simulink model "21-E"  (R2014a)
settings: Solver=FixedStepDiscrete  StartTime=0.0  StopTime=10.0  FixedStep=0.0005  RelTol=1e-3
undefined symbols (not defined in the file): add_k1_100, add_k2_100, ADDspeed, cal_acc_div, cal_acc_flo_add, cal_acc_min, cal_an_div, cal_an_min, cal_bre_div, cal_bre_en_add, cal_bre_flo_add, cal_bre_min, cal_conf_off, cal_conf_on, controller, ecucoder_acal, enres_on_add, enres_per_add
libraries: simulink x165, ec55xxlib x29
(part 5 of 6)

== system 21-E/run/ctrl/ECU_1L/ctrl_1L ==
  ctrl_1L : Inport
  BitCov : DataTypeConversion  OutDataTypeStr=uint8
  Constant{3..8} (6 alike) : Constant  Value=0  OutDataTypeStr=uint8
  ctrl_1LCOV : DataTypeConversion  OutDataTypeStr=uint8
  ctrl_1LRon : Rounding  Operator=round
  ctrl_1L_1sat : Saturate  UpperLimit=65535  LowerLimit=0
  ctrl_1L_And : simulink/Logic and Bit Operations/Bitwise Operator  logicop=AND  UseBitMask=off  NumInputPorts=2  BitMask=bin2dec('11011001')  BitMaskRealWorld=Stored Integer
  ctrl_1L_And_C : Constant  Value=255  OutDataTypeStr=uint32
  ctrl_1L_Convert : DataTypeConversion  OutDataTypeStr=uint32
  ctrl_1L_D : Product  Inputs=*/
  ctrl_1L_D1 : Product  Inputs=*/
  ctrl_1L_F : Constant  OutDataTypeStr=single
  ctrl_1L_L : simulink/Logic and Bit Operations/Bitwise Operator  logicop=AND  UseBitMask=on  BitMask=65535  BitMaskRealWorld=Stored Integer
  ctrl_1L_O : Constant  Value=0  OutDataTypeStr=single
  ctrl_1L_S : ArithShift
  ctrl_1L_sat : Saturate  UpperLimit=65535  LowerLimit=0
  ctrl_1L_st : Sum  Inputs=+-
  ctrl_1Loutput2_C : Constant  Value=256
  output1 : Outport
  output2 : Outport  Port=2
  output3 : Outport  Port=3
  output4 : Outport  Port=4
  output5 : Outport  Port=5
  output6 : Outport  Port=6
  output7 : Outport  Port=7
  output8 : Outport  Port=8
  wires:
  Constant8/1 -> output8/1
  Constant7/1 -> output7/1
  Constant6/1 -> output6/1
  Constant5/1 -> output5/1
  Constant4/1 -> output4/1
  Constant3/1 -> output3/1
  BitCov/1 -> output1/1
  ctrl_1L_And/1 -> BitCov/1
  ctrl_1L_And_C/1 -> ctrl_1L_And/2
  ctrl_1LCOV/1 -> output2/1
  ctrl_1L_D1/1 -> ctrl_1LCOV/1
  ctrl_1Loutput2_C/1 -> ctrl_1L_D1/2
  ctrl_1L_L/1 -> ctrl_1L_And/1, ctrl_1L_D1/1
  ctrl_1L_Convert/1 -> ctrl_1L_L/1
  ctrl_1L_1sat/1 -> ctrl_1L_Convert/1
  ctrl_1L_S/1 -> ctrl_1L_1sat/1
  ctrl_1LRon/1 -> ctrl_1L_S/1
  ctrl_1L_D/1 -> ctrl_1LRon/1
  ctrl_1L_F/1 -> ctrl_1L_D/2
  ctrl_1L_st/1 -> ctrl_1L_D/1
  ctrl_1L_O/1 -> ctrl_1L_st/2
  ctrl_1L_sat/1 -> ctrl_1L_st/1
  ctrl_1L/1 -> ctrl_1L_sat/1

== system 21-E/run/ctrl/ECU_1L/max_n ==
  max_n : Inport
  BitCov : DataTypeConversion  OutDataTypeStr=uint8
  Constant{1..2,5..8} (6 alike) : Constant  Value=0  OutDataTypeStr=uint8
  max_nABS : Abs
  max_nCOV : DataTypeConversion  OutDataTypeStr=uint8
  max_nCS : ArithShift  BitShiftNumber=-16
  max_nConS : Constant  OutDataTypeStr=single
  max_nCosR : Constant  Value=0  OutDataTypeStr=uint8
  max_nROP : RelationalOperator  Operator=<  OutDataTypeStr=boolean
  max_nRon : Rounding  Operator=round
  max_nSW : Switch  Criteria=u2 ~= 0
  max_n_1sat : Saturate  UpperLimit=65535  LowerLimit=0
  max_n_And : simulink/Logic and Bit Operations/Bitwise Operator  logicop=AND  UseBitMask=off  NumInputPorts=2  BitMask=bin2dec('11011001')  BitMaskRealWorld=Stored Integer
  max_n_And_C : Constant  Value=255  OutDataTypeStr=uint32
  max_n_Convert : DataTypeConversion  OutDataTypeStr=uint32
  max_n_D : Product  Inputs=*/
  max_n_D1 : Product  Inputs=*/
  max_n_F : Constant  OutDataTypeStr=single
  max_n_L : simulink/Logic and Bit Operations/Bitwise Operator  logicop=AND  UseBitMask=on  BitMask=65535  BitMaskRealWorld=Stored Integer
  max_n_O : Constant  Value=0  OutDataTypeStr=single
  max_n_S : ArithShift
  max_n_sat : Saturate  UpperLimit=32767  LowerLimit=-32768
  max_n_st : Sum  Inputs=+-
  max_noutput4_C : Constant  Value=256
  max_nsubcon : Sum  Inputs=+-
  output1 : Outport
  output2 : Outport  Port=2
  output3 : Outport  Port=3
  output4 : Outport  Port=4
  output5 : Outport  Port=5
  output6 : Outport  Port=6
  output7 : Outport  Port=7
  output8 : Outport  Port=8
  wires:
  Constant8/1 -> output8/1
  Constant7/1 -> output7/1
  Constant6/1 -> output6/1
  Constant5/1 -> output5/1
  Constant2/1 -> output2/1
  Constant1/1 -> output1/1
  BitCov/1 -> output3/1
  max_n_And/1 -> BitCov/1
  max_n_And_C/1 -> max_n_And/2
  max_nCOV/1 -> output4/1
  max_n_D1/1 -> max_nCOV/1
  max_noutput4_C/1 -> max_n_D1/2
  max_n_L/1 -> max_n_And/1, max_n_D1/1
  max_n_Convert/1 -> max_n_L/1
  max_n_1sat/1 -> max_n_Convert/1
  max_n_S/1 -> max_n_1sat/1
  max_nSW/1 -> max_n_S/1
  max_nROP/1 -> max_nSW/2
  max_nsubcon/1 -> max_nSW/1
  max_nABS/1 -> max_nsubcon/2
  max_nCS/1 -> max_nsubcon/1
  max_nConS/1 -> max_nCS/1
  max_nCosR/1 -> max_nROP/2
  max_nRon/1 -> max_nSW/3, max_nABS/1, max_nROP/1
  max_n_D/1 -> max_nRon/1
  max_n_F/1 -> max_n_D/2
  max_n_st/1 -> max_n_D/1
  max_n_O/1 -> max_n_st/2
  max_n_sat/1 -> max_n_st/1
  max_n/1 -> max_n_sat/1

== system 21-E/run/ctrl/ECU_1R/TN_1R ==
  TN_1R : Inport
  BitCov : DataTypeConversion  OutDataTypeStr=uint8
  Constant{1..6} (6 alike) : Constant  Value=0  OutDataTypeStr=uint8
  TN_1RABS : Abs
  TN_1RCOV : DataTypeConversion  OutDataTypeStr=uint8
  TN_1RCS : ArithShift  BitShiftNumber=-16
  TN_1RConS : Constant  OutDataTypeStr=single
  TN_1RCosR : Constant  Value=0  OutDataTypeStr=uint8
  TN_1RROP : RelationalOperator  Operator=<  OutDataTypeStr=boolean
  TN_1RRon : Rounding  Operator=round
  TN_1RSW : Switch  Criteria=u2 ~= 0
  TN_1R_1sat : Saturate  UpperLimit=65535  LowerLimit=0
  TN_1R_And : simulink/Logic and Bit Operations/Bitwise Operator  logicop=AND  UseBitMask=off  NumInputPorts=2  BitMask=bin2dec('11011001')  BitMaskRealWorld=Stored Integer
  TN_1R_And_C : Constant  Value=255  OutDataTypeStr=uint32
  TN_1R_Convert : DataTypeConversion  OutDataTypeStr=uint32
  TN_1R_D : Product  Inputs=*/
  TN_1R_D1 : Product  Inputs=*/
  TN_1R_F : Constant  OutDataTypeStr=single
  TN_1R_L : simulink/Logic and Bit Operations/Bitwise Operator  logicop=AND  UseBitMask=on  BitMask=65535  BitMaskRealWorld=Stored Integer
  TN_1R_O : Constant  Value=0  OutDataTypeStr=single
  TN_1R_S : ArithShift
  TN_1R_sat : Saturate  UpperLimit=32767  LowerLimit=-32768
  TN_1R_st : Sum  Inputs=+-
  TN_1Routput8_C : Constant  Value=256
  TN_1Rsubcon : Sum  Inputs=+-
  output1 : Outport
  output2 : Outport  Port=2
  output3 : Outport  Port=3
  output4 : Outport  Port=4
  output5 : Outport  Port=5
  output6 : Outport  Port=6
  output7 : Outport  Port=7
  output8 : Outport  Port=8
  wires:
  Constant6/1 -> output6/1
  Constant5/1 -> output5/1
  Constant4/1 -> output4/1
  Constant3/1 -> output3/1
  Constant2/1 -> output2/1
  Constant1/1 -> output1/1
  BitCov/1 -> output7/1
  TN_1R_And/1 -> BitCov/1
  TN_1R_And_C/1 -> TN_1R_And/2
  TN_1RCOV/1 -> output8/1
  TN_1R_D1/1 -> TN_1RCOV/1
  TN_1Routput8_C/1 -> TN_1R_D1/2
  TN_1R_L/1 -> TN_1R_And/1, TN_1R_D1/1
  TN_1R_Convert/1 -> TN_1R_L/1
  TN_1R_1sat/1 -> TN_1R_Convert/1
  TN_1R_S/1 -> TN_1R_1sat/1
  TN_1RSW/1 -> TN_1R_S/1
  TN_1RROP/1 -> TN_1RSW/2
  TN_1Rsubcon/1 -> TN_1RSW/1
  TN_1RABS/1 -> TN_1Rsubcon/2
  TN_1RCS/1 -> TN_1Rsubcon/1
  TN_1RConS/1 -> TN_1RCS/1
  TN_1RCosR/1 -> TN_1RROP/2
  TN_1RRon/1 -> TN_1RSW/3, TN_1RABS/1, TN_1RROP/1
  TN_1R_D/1 -> TN_1RRon/1
  TN_1R_F/1 -> TN_1R_D/2
  TN_1R_st/1 -> TN_1R_D/1
  TN_1R_O/1 -> TN_1R_st/2
  TN_1R_sat/1 -> TN_1R_st/1
  TN_1R/1 -> TN_1R_sat/1

== system 21-E/run/ctrl/ECU_1R/TP_1R ==
  TP_1R : Inport
  BitCov : DataTypeConversion  OutDataTypeStr=uint8
  Constant{1..4,7..8} (6 alike) : Constant  Value=0  OutDataTypeStr=uint8
  TP_1RABS : Abs
  TP_1RCOV : DataTypeConversion  OutDataTypeStr=uint8
  TP_1RCS : ArithShift  BitShiftNumber=-16
  TP_1RConS : Constant  OutDataTypeStr=single
  TP_1RCosR : Constant  Value=0  OutDataTypeStr=uint8
  TP_1RROP : RelationalOperator  Operator=<  OutDataTypeStr=boolean
  TP_1RRon : Rounding  Operator=round
  TP_1RSW : Switch  Criteria=u2 ~= 0
  TP_1R_1sat : Saturate  UpperLimit=65535  LowerLimit=0
  TP_1R_And : simulink/Logic and Bit Operations/Bitwise Operator  logicop=AND  UseBitMask=off  NumInputPorts=2  BitMask=bin2dec('11011001')  BitMaskRealWorld=Stored Integer
  TP_1R_And_C : Constant  Value=255  OutDataTypeStr=uint32
  TP_1R_Convert : DataTypeConversion  OutDataTypeStr=uint32
  TP_1R_D : Product  Inputs=*/
  TP_1R_D1 : Product  Inputs=*/
  TP_1R_F : Constant  OutDataTypeStr=single
  TP_1R_L : simulink/Logic and Bit Operations/Bitwise Operator  logicop=AND  UseBitMask=on  BitMask=65535  BitMaskRealWorld=Stored Integer
  TP_1R_O : Constant  Value=0  OutDataTypeStr=single
  TP_1R_S : ArithShift
  TP_1R_sat : Saturate  UpperLimit=32767  LowerLimit=-32768
  TP_1R_st : Sum  Inputs=+-
  TP_1Routput6_C : Constant  Value=256
  TP_1Rsubcon : Sum  Inputs=+-
  output1 : Outport
  output2 : Outport  Port=2
  output3 : Outport  Port=3
  output4 : Outport  Port=4
  output5 : Outport  Port=5
  output6 : Outport  Port=6
  output7 : Outport  Port=7
  output8 : Outport  Port=8
  wires:
  Constant8/1 -> output8/1
  Constant7/1 -> output7/1
  Constant4/1 -> output4/1
  Constant3/1 -> output3/1
  Constant2/1 -> output2/1
  Constant1/1 -> output1/1
  BitCov/1 -> output5/1
  TP_1R_And/1 -> BitCov/1
  TP_1R_And_C/1 -> TP_1R_And/2
  TP_1RCOV/1 -> output6/1
  TP_1R_D1/1 -> TP_1RCOV/1
  TP_1Routput6_C/1 -> TP_1R_D1/2
  TP_1R_L/1 -> TP_1R_And/1, TP_1R_D1/1
  TP_1R_Convert/1 -> TP_1R_L/1
  TP_1R_1sat/1 -> TP_1R_Convert/1
  TP_1R_S/1 -> TP_1R_1sat/1
  TP_1RSW/1 -> TP_1R_S/1
  TP_1RROP/1 -> TP_1RSW/2
  TP_1Rsubcon/1 -> TP_1RSW/1
  TP_1RABS/1 -> TP_1Rsubcon/2
  TP_1RCS/1 -> TP_1Rsubcon/1
  TP_1RConS/1 -> TP_1RCS/1
  TP_1RCosR/1 -> TP_1RROP/2
  TP_1RRon/1 -> TP_1RSW/3, TP_1RABS/1, TP_1RROP/1
  TP_1R_D/1 -> TP_1RRon/1
  TP_1R_F/1 -> TP_1R_D/2
  TP_1R_st/1 -> TP_1R_D/1
  TP_1R_O/1 -> TP_1R_st/2
  TP_1R_sat/1 -> TP_1R_st/1
  TP_1R/1 -> TP_1R_sat/1

== system 21-E/run/ctrl/ECU_1R/ctrl_1R ==
  ctrl_1R : Inport
  BitCov : DataTypeConversion  OutDataTypeStr=uint8
  Constant{3..8} (6 alike) : Constant  Value=0  OutDataTypeStr=uint8
  ctrl_1RCOV : DataTypeConversion  OutDataTypeStr=uint8
  ctrl_1RRon : Rounding  Operator=round
  ctrl_1R_1sat : Saturate  UpperLimit=65535  LowerLimit=0
  ctrl_1R_And : simulink/Logic and Bit Operations/Bitwise Operator  logicop=AND  UseBitMask=off  NumInputPorts=2  BitMask=bin2dec('11011001')  BitMaskRealWorld=Stored Integer
  ctrl_1R_And_C : Constant  Value=255  OutDataTypeStr=uint32
  ctrl_1R_Convert : DataTypeConversion  OutDataTypeStr=uint32
  ctrl_1R_D : Product  Inputs=*/
  ctrl_1R_D1 : Product  Inputs=*/
  ctrl_1R_F : Constant  OutDataTypeStr=single
  ctrl_1R_L : simulink/Logic and Bit Operations/Bitwise Operator  logicop=AND  UseBitMask=on  BitMask=65535  BitMaskRealWorld=Stored Integer
  ctrl_1R_O : Constant  Value=0  OutDataTypeStr=single
  ctrl_1R_S : ArithShift
  ctrl_1R_sat : Saturate  UpperLimit=65535  LowerLimit=0
  ctrl_1R_st : Sum  Inputs=+-
  ctrl_1Routput2_C : Constant  Value=256
  output1 : Outport
  output2 : Outport  Port=2
  output3 : Outport  Port=3
  output4 : Outport  Port=4
  output5 : Outport  Port=5
  output6 : Outport  Port=6
  output7 : Outport  Port=7
  output8 : Outport  Port=8
  wires:
  Constant8/1 -> output8/1
  Constant7/1 -> output7/1
  Constant6/1 -> output6/1
  Constant5/1 -> output5/1
  Constant4/1 -> output4/1
  Constant3/1 -> output3/1
  BitCov/1 -> output1/1
  ctrl_1R_And/1 -> BitCov/1
  ctrl_1R_And_C/1 -> ctrl_1R_And/2
  ctrl_1RCOV/1 -> output2/1
  ctrl_1R_D1/1 -> ctrl_1RCOV/1
  ctrl_1Routput2_C/1 -> ctrl_1R_D1/2
  ctrl_1R_L/1 -> ctrl_1R_And/1, ctrl_1R_D1/1
  ctrl_1R_Convert/1 -> ctrl_1R_L/1
  ctrl_1R_1sat/1 -> ctrl_1R_Convert/1
  ctrl_1R_S/1 -> ctrl_1R_1sat/1
  ctrl_1RRon/1 -> ctrl_1R_S/1
  ctrl_1R_D/1 -> ctrl_1RRon/1
  ctrl_1R_F/1 -> ctrl_1R_D/2
  ctrl_1R_st/1 -> ctrl_1R_D/1
  ctrl_1R_O/1 -> ctrl_1R_st/2
  ctrl_1R_sat/1 -> ctrl_1R_st/1
  ctrl_1R/1 -> ctrl_1R_sat/1

== system 21-E/run/ctrl/ECU_1R/max_n ==
  max_n : Inport
  BitCov : DataTypeConversion  OutDataTypeStr=uint8
  Constant{1..2,5..8} (6 alike) : Constant  Value=0  OutDataTypeStr=uint8
  max_nABS : Abs
  max_nCOV : DataTypeConversion  OutDataTypeStr=uint8
  max_nCS : ArithShift  BitShiftNumber=-16
  max_nConS : Constant  OutDataTypeStr=single
  max_nCosR : Constant  Value=0  OutDataTypeStr=uint8
  max_nROP : RelationalOperator  Operator=<  OutDataTypeStr=boolean
  max_nRon : Rounding  Operator=round
  max_nSW : Switch  Criteria=u2 ~= 0
  max_n_1sat : Saturate  UpperLimit=65535  LowerLimit=0
  max_n_And : simulink/Logic and Bit Operations/Bitwise Operator  logicop=AND  UseBitMask=off  NumInputPorts=2  BitMask=bin2dec('11011001')  BitMaskRealWorld=Stored Integer
  max_n_And_C : Constant  Value=255  OutDataTypeStr=uint32
  max_n_Convert : DataTypeConversion  OutDataTypeStr=uint32
  max_n_D : Product  Inputs=*/
  max_n_D1 : Product  Inputs=*/
  max_n_F : Constant  OutDataTypeStr=single
  max_n_L : simulink/Logic and Bit Operations/Bitwise Operator  logicop=AND  UseBitMask=on  BitMask=65535  BitMaskRealWorld=Stored Integer
  max_n_O : Constant  Value=0  OutDataTypeStr=single
  max_n_S : ArithShift
  max_n_sat : Saturate  UpperLimit=32767  LowerLimit=-32768
  max_n_st : Sum  Inputs=+-
  max_noutput4_C : Constant  Value=256
  max_nsubcon : Sum  Inputs=+-
  output1 : Outport
  output2 : Outport  Port=2
  output3 : Outport  Port=3
  output4 : Outport  Port=4
  output5 : Outport  Port=5
  output6 : Outport  Port=6
  output7 : Outport  Port=7
  output8 : Outport  Port=8
  wires:
  Constant8/1 -> output8/1
  Constant7/1 -> output7/1
  Constant6/1 -> output6/1
  Constant5/1 -> output5/1
  Constant2/1 -> output2/1
  Constant1/1 -> output1/1
  BitCov/1 -> output3/1
  max_n_And/1 -> BitCov/1
  max_n_And_C/1 -> max_n_And/2
  max_nCOV/1 -> output4/1
  max_n_D1/1 -> max_nCOV/1
  max_noutput4_C/1 -> max_n_D1/2
  max_n_L/1 -> max_n_And/1, max_n_D1/1
  max_n_Convert/1 -> max_n_L/1
  max_n_1sat/1 -> max_n_Convert/1
  max_n_S/1 -> max_n_1sat/1
  max_nSW/1 -> max_n_S/1
  max_nROP/1 -> max_nSW/2
  max_nsubcon/1 -> max_nSW/1
  max_nABS/1 -> max_nsubcon/2
  max_nCS/1 -> max_nsubcon/1
  max_nConS/1 -> max_nCS/1
  max_nCosR/1 -> max_nROP/2
  max_nRon/1 -> max_nSW/3, max_nABS/1, max_nROP/1
  max_n_D/1 -> max_nRon/1
  max_n_F/1 -> max_n_D/2
  max_n_st/1 -> max_n_D/1
  max_n_O/1 -> max_n_st/2
  max_n_sat/1 -> max_n_st/1
  max_n/1 -> max_n_sat/1

== system 21-E/run/ctrl/ECU_2L/TN_2L ==
  TN_2L : Inport
  BitCov : DataTypeConversion  OutDataTypeStr=uint8
  Constant{1..6} (6 alike) : Constant  Value=0  OutDataTypeStr=uint8
  TN_2LABS : Abs
  TN_2LCOV : DataTypeConversion  OutDataTypeStr=uint8
  TN_2LCS : ArithShift  BitShiftNumber=-16
  TN_2LConS : Constant  OutDataTypeStr=single
  TN_2LCosR : Constant  Value=0  OutDataTypeStr=uint8
  TN_2LROP : RelationalOperator  Operator=<  OutDataTypeStr=boolean
  TN_2LRon : Rounding  Operator=round
  TN_2LSW : Switch  Criteria=u2 ~= 0
  TN_2L_1sat : Saturate  UpperLimit=65535  LowerLimit=0
  TN_2L_And : simulink/Logic and Bit Operations/Bitwise Operator  logicop=AND  UseBitMask=off  NumInputPorts=2  BitMask=bin2dec('11011001')  BitMaskRealWorld=Stored Integer
  TN_2L_And_C : Constant  Value=255  OutDataTypeStr=uint32
  TN_2L_Convert : DataTypeConversion  OutDataTypeStr=uint32
  TN_2L_D : Product  Inputs=*/
  TN_2L_D1 : Product  Inputs=*/
  TN_2L_F : Constant  OutDataTypeStr=single
  TN_2L_L : simulink/Logic and Bit Operations/Bitwise Operator  logicop=AND  UseBitMask=on  BitMask=65535  BitMaskRealWorld=Stored Integer
  TN_2L_O : Constant  Value=0  OutDataTypeStr=single
  TN_2L_S : ArithShift
  TN_2L_sat : Saturate  UpperLimit=32767  LowerLimit=-32768
  TN_2L_st : Sum  Inputs=+-
  TN_2Loutput8_C : Constant  Value=256
  TN_2Lsubcon : Sum  Inputs=+-
  output1 : Outport
  output2 : Outport  Port=2
  output3 : Outport  Port=3
  output4 : Outport  Port=4
  output5 : Outport  Port=5
  output6 : Outport  Port=6
  output7 : Outport  Port=7
  output8 : Outport  Port=8
  wires:
  Constant6/1 -> output6/1
  Constant5/1 -> output5/1
  Constant4/1 -> output4/1
  Constant3/1 -> output3/1
  Constant2/1 -> output2/1
  Constant1/1 -> output1/1
  BitCov/1 -> output7/1
  TN_2L_And/1 -> BitCov/1
  TN_2L_And_C/1 -> TN_2L_And/2
  TN_2LCOV/1 -> output8/1
  TN_2L_D1/1 -> TN_2LCOV/1
  TN_2Loutput8_C/1 -> TN_2L_D1/2
  TN_2L_L/1 -> TN_2L_And/1, TN_2L_D1/1
  TN_2L_Convert/1 -> TN_2L_L/1
  TN_2L_1sat/1 -> TN_2L_Convert/1
  TN_2L_S/1 -> TN_2L_1sat/1
  TN_2LSW/1 -> TN_2L_S/1
  TN_2LROP/1 -> TN_2LSW/2
  TN_2Lsubcon/1 -> TN_2LSW/1
  TN_2LABS/1 -> TN_2Lsubcon/2
  TN_2LCS/1 -> TN_2Lsubcon/1
  TN_2LConS/1 -> TN_2LCS/1
  TN_2LCosR/1 -> TN_2LROP/2
  TN_2LRon/1 -> TN_2LSW/3, TN_2LABS/1, TN_2LROP/1
  TN_2L_D/1 -> TN_2LRon/1
  TN_2L_F/1 -> TN_2L_D/2
  TN_2L_st/1 -> TN_2L_D/1
  TN_2L_O/1 -> TN_2L_st/2
  TN_2L_sat/1 -> TN_2L_st/1
  TN_2L/1 -> TN_2L_sat/1

== system 21-E/run/ctrl/ECU_2L/TP_2L ==
  TP_2L : Inport
  BitCov : DataTypeConversion  OutDataTypeStr=uint8
  Constant{1..4,7..8} (6 alike) : Constant  Value=0  OutDataTypeStr=uint8
  TP_2LABS : Abs
  TP_2LCOV : DataTypeConversion  OutDataTypeStr=uint8
  TP_2LCS : ArithShift  BitShiftNumber=-16
  TP_2LConS : Constant  OutDataTypeStr=single
  TP_2LCosR : Constant  Value=0  OutDataTypeStr=uint8
  TP_2LROP : RelationalOperator  Operator=<  OutDataTypeStr=boolean
  TP_2LRon : Rounding  Operator=round
  TP_2LSW : Switch  Criteria=u2 ~= 0
  TP_2L_1sat : Saturate  UpperLimit=65535  LowerLimit=0
  TP_2L_And : simulink/Logic and Bit Operations/Bitwise Operator  logicop=AND  UseBitMask=off  NumInputPorts=2  BitMask=bin2dec('11011001')  BitMaskRealWorld=Stored Integer
  TP_2L_And_C : Constant  Value=255  OutDataTypeStr=uint32
  TP_2L_Convert : DataTypeConversion  OutDataTypeStr=uint32
  TP_2L_D : Product  Inputs=*/
  TP_2L_D1 : Product  Inputs=*/
  TP_2L_F : Constant  OutDataTypeStr=single
  TP_2L_L : simulink/Logic and Bit Operations/Bitwise Operator  logicop=AND  UseBitMask=on  BitMask=65535  BitMaskRealWorld=Stored Integer
  TP_2L_O : Constant  Value=0  OutDataTypeStr=single
  TP_2L_S : ArithShift
  TP_2L_sat : Saturate  UpperLimit=32767  LowerLimit=-32768
  TP_2L_st : Sum  Inputs=+-
  TP_2Loutput6_C : Constant  Value=256
  TP_2Lsubcon : Sum  Inputs=+-
  output1 : Outport
  output2 : Outport  Port=2
  output3 : Outport  Port=3
  output4 : Outport  Port=4
  output5 : Outport  Port=5
  output6 : Outport  Port=6
  output7 : Outport  Port=7
  output8 : Outport  Port=8
  wires:
  Constant8/1 -> output8/1
  Constant7/1 -> output7/1
  Constant4/1 -> output4/1
  Constant3/1 -> output3/1
  Constant2/1 -> output2/1
  Constant1/1 -> output1/1
  BitCov/1 -> output5/1
  TP_2L_And/1 -> BitCov/1
  TP_2L_And_C/1 -> TP_2L_And/2
  TP_2LCOV/1 -> output6/1
  TP_2L_D1/1 -> TP_2LCOV/1
  TP_2Loutput6_C/1 -> TP_2L_D1/2
  TP_2L_L/1 -> TP_2L_And/1, TP_2L_D1/1
  TP_2L_Convert/1 -> TP_2L_L/1
  TP_2L_1sat/1 -> TP_2L_Convert/1
  TP_2L_S/1 -> TP_2L_1sat/1
  TP_2LSW/1 -> TP_2L_S/1
  TP_2LROP/1 -> TP_2LSW/2
  TP_2Lsubcon/1 -> TP_2LSW/1
  TP_2LABS/1 -> TP_2Lsubcon/2
  TP_2LCS/1 -> TP_2Lsubcon/1
  TP_2LConS/1 -> TP_2LCS/1
  TP_2LCosR/1 -> TP_2LROP/2
  TP_2LRon/1 -> TP_2LSW/3, TP_2LABS/1, TP_2LROP/1
  TP_2L_D/1 -> TP_2LRon/1
  TP_2L_F/1 -> TP_2L_D/2
  TP_2L_st/1 -> TP_2L_D/1
  TP_2L_O/1 -> TP_2L_st/2
  TP_2L_sat/1 -> TP_2L_st/1
  TP_2L/1 -> TP_2L_sat/1

== system 21-E/run/ctrl/ECU_2L/ctrl_2L ==
  ctrl_2L : Inport
  BitCov : DataTypeConversion  OutDataTypeStr=uint8
  Constant{3..8} (6 alike) : Constant  Value=0  OutDataTypeStr=uint8
  ctrl_2LCOV : DataTypeConversion  OutDataTypeStr=uint8
  ctrl_2LRon : Rounding  Operator=round
  ctrl_2L_1sat : Saturate  UpperLimit=65535  LowerLimit=0
  ctrl_2L_And : simulink/Logic and Bit Operations/Bitwise Operator  logicop=AND  UseBitMask=off  NumInputPorts=2  BitMask=bin2dec('11011001')  BitMaskRealWorld=Stored Integer
  ctrl_2L_And_C : Constant  Value=255  OutDataTypeStr=uint32
  ctrl_2L_Convert : DataTypeConversion  OutDataTypeStr=uint32
  ctrl_2L_D : Product  Inputs=*/
  ctrl_2L_D1 : Product  Inputs=*/
  ctrl_2L_F : Constant  OutDataTypeStr=single
  ctrl_2L_L : simulink/Logic and Bit Operations/Bitwise Operator  logicop=AND  UseBitMask=on  BitMask=65535  BitMaskRealWorld=Stored Integer
  ctrl_2L_O : Constant  Value=0  OutDataTypeStr=single
  ctrl_2L_S : ArithShift
  ctrl_2L_sat : Saturate  UpperLimit=65535  LowerLimit=0
  ctrl_2L_st : Sum  Inputs=+-
  ctrl_2Loutput2_C : Constant  Value=256
  output1 : Outport
  output2 : Outport  Port=2
  output3 : Outport  Port=3
  output4 : Outport  Port=4
  output5 : Outport  Port=5
  output6 : Outport  Port=6
  output7 : Outport  Port=7
  output8 : Outport  Port=8
  wires:
  Constant8/1 -> output8/1
  Constant7/1 -> output7/1
  Constant6/1 -> output6/1
  Constant5/1 -> output5/1
  Constant4/1 -> output4/1
  Constant3/1 -> output3/1
  BitCov/1 -> output1/1
  ctrl_2L_And/1 -> BitCov/1
  ctrl_2L_And_C/1 -> ctrl_2L_And/2
  ctrl_2LCOV/1 -> output2/1
  ctrl_2L_D1/1 -> ctrl_2LCOV/1
  ctrl_2Loutput2_C/1 -> ctrl_2L_D1/2
  ctrl_2L_L/1 -> ctrl_2L_And/1, ctrl_2L_D1/1
  ctrl_2L_Convert/1 -> ctrl_2L_L/1
  ctrl_2L_1sat/1 -> ctrl_2L_Convert/1
  ctrl_2L_S/1 -> ctrl_2L_1sat/1
  ctrl_2LRon/1 -> ctrl_2L_S/1
  ctrl_2L_D/1 -> ctrl_2LRon/1
  ctrl_2L_F/1 -> ctrl_2L_D/2
  ctrl_2L_st/1 -> ctrl_2L_D/1
  ctrl_2L_O/1 -> ctrl_2L_st/2
  ctrl_2L_sat/1 -> ctrl_2L_st/1
  ctrl_2L/1 -> ctrl_2L_sat/1

== system 21-E/run/ctrl/ECU_2L/max_n ==
  max_n : Inport
  BitCov : DataTypeConversion  OutDataTypeStr=uint8
  Constant{1..2,5..8} (6 alike) : Constant  Value=0  OutDataTypeStr=uint8
  max_nABS : Abs
  max_nCOV : DataTypeConversion  OutDataTypeStr=uint8
  max_nCS : ArithShift  BitShiftNumber=-16
  max_nConS : Constant  OutDataTypeStr=single
  max_nCosR : Constant  Value=0  OutDataTypeStr=uint8
  max_nROP : RelationalOperator  Operator=<  OutDataTypeStr=boolean
  max_nRon : Rounding  Operator=round
  max_nSW : Switch  Criteria=u2 ~= 0
  max_n_1sat : Saturate  UpperLimit=65535  LowerLimit=0
  max_n_And : simulink/Logic and Bit Operations/Bitwise Operator  logicop=AND  UseBitMask=off  NumInputPorts=2  BitMask=bin2dec('11011001')  BitMaskRealWorld=Stored Integer
  max_n_And_C : Constant  Value=255  OutDataTypeStr=uint32
  max_n_Convert : DataTypeConversion  OutDataTypeStr=uint32
  max_n_D : Product  Inputs=*/
  max_n_D1 : Product  Inputs=*/
  max_n_F : Constant  OutDataTypeStr=single
  max_n_L : simulink/Logic and Bit Operations/Bitwise Operator  logicop=AND  UseBitMask=on  BitMask=65535  BitMaskRealWorld=Stored Integer
  max_n_O : Constant  Value=0  OutDataTypeStr=single
  max_n_S : ArithShift
  max_n_sat : Saturate  UpperLimit=32767  LowerLimit=-32768
  max_n_st : Sum  Inputs=+-
  max_noutput4_C : Constant  Value=256
  max_nsubcon : Sum  Inputs=+-
  output1 : Outport
  output2 : Outport  Port=2
  output3 : Outport  Port=3
  output4 : Outport  Port=4
  output5 : Outport  Port=5
  output6 : Outport  Port=6
  output7 : Outport  Port=7
  output8 : Outport  Port=8
  wires:
  Constant8/1 -> output8/1
  Constant7/1 -> output7/1
  Constant6/1 -> output6/1
  Constant5/1 -> output5/1
  Constant2/1 -> output2/1
  Constant1/1 -> output1/1
  BitCov/1 -> output3/1
  max_n_And/1 -> BitCov/1
  max_n_And_C/1 -> max_n_And/2
  max_nCOV/1 -> output4/1
  max_n_D1/1 -> max_nCOV/1
  max_noutput4_C/1 -> max_n_D1/2
  max_n_L/1 -> max_n_And/1, max_n_D1/1
  max_n_Convert/1 -> max_n_L/1
  max_n_1sat/1 -> max_n_Convert/1
  max_n_S/1 -> max_n_1sat/1
  max_nSW/1 -> max_n_S/1
  max_nROP/1 -> max_nSW/2
  max_nsubcon/1 -> max_nSW/1
  max_nABS/1 -> max_nsubcon/2
  max_nCS/1 -> max_nsubcon/1
  max_nConS/1 -> max_nCS/1
  max_nCosR/1 -> max_nROP/2
  max_nRon/1 -> max_nSW/3, max_nABS/1, max_nROP/1
  max_n_D/1 -> max_nRon/1
  max_n_F/1 -> max_n_D/2
  max_n_st/1 -> max_n_D/1
  max_n_O/1 -> max_n_st/2
  max_n_sat/1 -> max_n_st/1
  max_n/1 -> max_n_sat/1

== system 21-E/run/ctrl/ECU_2R/TN_2R ==
  TN_2R : Inport
  BitCov : DataTypeConversion  OutDataTypeStr=uint8
  Constant{1..6} (6 alike) : Constant  Value=0  OutDataTypeStr=uint8
  TN_2RABS : Abs
  TN_2RCOV : DataTypeConversion  OutDataTypeStr=uint8
  TN_2RCS : ArithShift  BitShiftNumber=-16
  TN_2RConS : Constant  OutDataTypeStr=single
  TN_2RCosR : Constant  Value=0  OutDataTypeStr=uint8
  TN_2RROP : RelationalOperator  Operator=<  OutDataTypeStr=boolean
  TN_2RRon : Rounding  Operator=round
  TN_2RSW : Switch  Criteria=u2 ~= 0
  TN_2R_1sat : Saturate  UpperLimit=65535  LowerLimit=0
  TN_2R_And : simulink/Logic and Bit Operations/Bitwise Operator  logicop=AND  UseBitMask=off  NumInputPorts=2  BitMask=bin2dec('11011001')  BitMaskRealWorld=Stored Integer
  TN_2R_And_C : Constant  Value=255  OutDataTypeStr=uint32
  TN_2R_Convert : DataTypeConversion  OutDataTypeStr=uint32
  TN_2R_D : Product  Inputs=*/
  TN_2R_D1 : Product  Inputs=*/
  TN_2R_F : Constant  OutDataTypeStr=single
  TN_2R_L : simulink/Logic and Bit Operations/Bitwise Operator  logicop=AND  UseBitMask=on  BitMask=65535  BitMaskRealWorld=Stored Integer
  TN_2R_O : Constant  Value=0  OutDataTypeStr=single
  TN_2R_S : ArithShift
  TN_2R_sat : Saturate  UpperLimit=32767  LowerLimit=-32768
  TN_2R_st : Sum  Inputs=+-
  TN_2Routput8_C : Constant  Value=256
  TN_2Rsubcon : Sum  Inputs=+-
  output1 : Outport
  output2 : Outport  Port=2
  output3 : Outport  Port=3
  output4 : Outport  Port=4
  output5 : Outport  Port=5
  output6 : Outport  Port=6
  output7 : Outport  Port=7
  output8 : Outport  Port=8
  wires:
  Constant6/1 -> output6/1
  Constant5/1 -> output5/1
  Constant4/1 -> output4/1
  Constant3/1 -> output3/1
  Constant2/1 -> output2/1
  Constant1/1 -> output1/1
  BitCov/1 -> output7/1
  TN_2R_And/1 -> BitCov/1
  TN_2R_And_C/1 -> TN_2R_And/2
  TN_2RCOV/1 -> output8/1
  TN_2R_D1/1 -> TN_2RCOV/1
  TN_2Routput8_C/1 -> TN_2R_D1/2
  TN_2R_L/1 -> TN_2R_And/1, TN_2R_D1/1
  TN_2R_Convert/1 -> TN_2R_L/1
  TN_2R_1sat/1 -> TN_2R_Convert/1
  TN_2R_S/1 -> TN_2R_1sat/1
  TN_2RSW/1 -> TN_2R_S/1
  TN_2RROP/1 -> TN_2RSW/2
  TN_2Rsubcon/1 -> TN_2RSW/1
  TN_2RABS/1 -> TN_2Rsubcon/2
  TN_2RCS/1 -> TN_2Rsubcon/1
  TN_2RConS/1 -> TN_2RCS/1
  TN_2RCosR/1 -> TN_2RROP/2
  TN_2RRon/1 -> TN_2RSW/3, TN_2RABS/1, TN_2RROP/1
  TN_2R_D/1 -> TN_2RRon/1
  TN_2R_F/1 -> TN_2R_D/2
  TN_2R_st/1 -> TN_2R_D/1
  TN_2R_O/1 -> TN_2R_st/2
  TN_2R_sat/1 -> TN_2R_st/1
  TN_2R/1 -> TN_2R_sat/1

== system 21-E/run/ctrl/ECU_2R/TP_2R ==
  TP_2R : Inport
  BitCov : DataTypeConversion  OutDataTypeStr=uint8
  Constant{1..4,7..8} (6 alike) : Constant  Value=0  OutDataTypeStr=uint8
  TP_2RABS : Abs
  TP_2RCOV : DataTypeConversion  OutDataTypeStr=uint8
  TP_2RCS : ArithShift  BitShiftNumber=-16
  TP_2RConS : Constant  OutDataTypeStr=single
  TP_2RCosR : Constant  Value=0  OutDataTypeStr=uint8
  TP_2RROP : RelationalOperator  Operator=<  OutDataTypeStr=boolean
  TP_2RRon : Rounding  Operator=round
  TP_2RSW : Switch  Criteria=u2 ~= 0
  TP_2R_1sat : Saturate  UpperLimit=65535  LowerLimit=0
  TP_2R_And : simulink/Logic and Bit Operations/Bitwise Operator  logicop=AND  UseBitMask=off  NumInputPorts=2  BitMask=bin2dec('11011001')  BitMaskRealWorld=Stored Integer
  TP_2R_And_C : Constant  Value=255  OutDataTypeStr=uint32
  TP_2R_Convert : DataTypeConversion  OutDataTypeStr=uint32
  TP_2R_D : Product  Inputs=*/
  TP_2R_D1 : Product  Inputs=*/
  TP_2R_F : Constant  OutDataTypeStr=single
  TP_2R_L : simulink/Logic and Bit Operations/Bitwise Operator  logicop=AND  UseBitMask=on  BitMask=65535  BitMaskRealWorld=Stored Integer
  TP_2R_O : Constant  Value=0  OutDataTypeStr=single
  TP_2R_S : ArithShift
  TP_2R_sat : Saturate  UpperLimit=32767  LowerLimit=-32768
  TP_2R_st : Sum  Inputs=+-
  TP_2Routput6_C : Constant  Value=256
  TP_2Rsubcon : Sum  Inputs=+-
  output1 : Outport
  output2 : Outport  Port=2
  output3 : Outport  Port=3
  output4 : Outport  Port=4
  output5 : Outport  Port=5
  output6 : Outport  Port=6
  output7 : Outport  Port=7
  output8 : Outport  Port=8
  wires:
  Constant8/1 -> output8/1
  Constant7/1 -> output7/1
  Constant4/1 -> output4/1
  Constant3/1 -> output3/1
  Constant2/1 -> output2/1
  Constant1/1 -> output1/1
  BitCov/1 -> output5/1
  TP_2R_And/1 -> BitCov/1
  TP_2R_And_C/1 -> TP_2R_And/2
  TP_2RCOV/1 -> output6/1
  TP_2R_D1/1 -> TP_2RCOV/1
  TP_2Routput6_C/1 -> TP_2R_D1/2
  TP_2R_L/1 -> TP_2R_And/1, TP_2R_D1/1
  TP_2R_Convert/1 -> TP_2R_L/1
  TP_2R_1sat/1 -> TP_2R_Convert/1
  TP_2R_S/1 -> TP_2R_1sat/1
  TP_2RSW/1 -> TP_2R_S/1
  TP_2RROP/1 -> TP_2RSW/2
  TP_2Rsubcon/1 -> TP_2RSW/1
  TP_2RABS/1 -> TP_2Rsubcon/2
  TP_2RCS/1 -> TP_2Rsubcon/1
  TP_2RConS/1 -> TP_2RCS/1
  TP_2RCosR/1 -> TP_2RROP/2
  TP_2RRon/1 -> TP_2RSW/3, TP_2RABS/1, TP_2RROP/1
  TP_2R_D/1 -> TP_2RRon/1
  TP_2R_F/1 -> TP_2R_D/2
  TP_2R_st/1 -> TP_2R_D/1
  TP_2R_O/1 -> TP_2R_st/2
  TP_2R_sat/1 -> TP_2R_st/1
  TP_2R/1 -> TP_2R_sat/1

== system 21-E/run/ctrl/ECU_2R/ctrl_2R ==
  ctrl_2R : Inport
  BitCov : DataTypeConversion  OutDataTypeStr=uint8
  Constant{3..8} (6 alike) : Constant  Value=0  OutDataTypeStr=uint8
  ctrl_2RCOV : DataTypeConversion  OutDataTypeStr=uint8
  ctrl_2RRon : Rounding  Operator=round
  ctrl_2R_1sat : Saturate  UpperLimit=65535  LowerLimit=0
  ctrl_2R_And : simulink/Logic and Bit Operations/Bitwise Operator  logicop=AND  UseBitMask=off  NumInputPorts=2  BitMask=bin2dec('11011001')  BitMaskRealWorld=Stored Integer
  ctrl_2R_And_C : Constant  Value=255  OutDataTypeStr=uint32
  ctrl_2R_Convert : DataTypeConversion  OutDataTypeStr=uint32
  ctrl_2R_D : Product  Inputs=*/
  ctrl_2R_D1 : Product  Inputs=*/
  ctrl_2R_F : Constant  OutDataTypeStr=single
  ctrl_2R_L : simulink/Logic and Bit Operations/Bitwise Operator  logicop=AND  UseBitMask=on  BitMask=65535  BitMaskRealWorld=Stored Integer
  ctrl_2R_O : Constant  Value=0  OutDataTypeStr=single
  ctrl_2R_S : ArithShift
  ctrl_2R_sat : Saturate  UpperLimit=65535  LowerLimit=0
  ctrl_2R_st : Sum  Inputs=+-
  ctrl_2Routput2_C : Constant  Value=256
  output1 : Outport
  output2 : Outport  Port=2
  output3 : Outport  Port=3
  output4 : Outport  Port=4
  output5 : Outport  Port=5
  output6 : Outport  Port=6
  output7 : Outport  Port=7
  output8 : Outport  Port=8
  wires:
  Constant8/1 -> output8/1
  Constant7/1 -> output7/1
  Constant6/1 -> output6/1
  Constant5/1 -> output5/1
  Constant4/1 -> output4/1
  Constant3/1 -> output3/1
  BitCov/1 -> output1/1
  ctrl_2R_And/1 -> BitCov/1
  ctrl_2R_And_C/1 -> ctrl_2R_And/2
  ctrl_2RCOV/1 -> output2/1
  ctrl_2R_D1/1 -> ctrl_2RCOV/1
  ctrl_2Routput2_C/1 -> ctrl_2R_D1/2
  ctrl_2R_L/1 -> ctrl_2R_And/1, ctrl_2R_D1/1
  ctrl_2R_Convert/1 -> ctrl_2R_L/1
  ctrl_2R_1sat/1 -> ctrl_2R_Convert/1
  ctrl_2R_S/1 -> ctrl_2R_1sat/1
  ctrl_2RRon/1 -> ctrl_2R_S/1
  ctrl_2R_D/1 -> ctrl_2RRon/1
  ctrl_2R_F/1 -> ctrl_2R_D/2
  ctrl_2R_st/1 -> ctrl_2R_D/1
  ctrl_2R_O/1 -> ctrl_2R_st/2
  ctrl_2R_sat/1 -> ctrl_2R_st/1
  ctrl_2R/1 -> ctrl_2R_sat/1

== system 21-E/run/ctrl/ECU_2R/max_n ==
  max_n : Inport
  BitCov : DataTypeConversion  OutDataTypeStr=uint8
  Constant{1..2,5..8} (6 alike) : Constant  Value=0  OutDataTypeStr=uint8
  max_nABS : Abs
  max_nCOV : DataTypeConversion  OutDataTypeStr=uint8
  max_nCS : ArithShift  BitShiftNumber=-16
  max_nConS : Constant  OutDataTypeStr=single
  max_nCosR : Constant  Value=0  OutDataTypeStr=uint8
  max_nROP : RelationalOperator  Operator=<  OutDataTypeStr=boolean
  max_nRon : Rounding  Operator=round
  max_nSW : Switch  Criteria=u2 ~= 0
  max_n_1sat : Saturate  UpperLimit=65535  LowerLimit=0
  max_n_And : simulink/Logic and Bit Operations/Bitwise Operator  logicop=AND  UseBitMask=off  NumInputPorts=2  BitMask=bin2dec('11011001')  BitMaskRealWorld=Stored Integer
  max_n_And_C : Constant  Value=255  OutDataTypeStr=uint32
  max_n_Convert : DataTypeConversion  OutDataTypeStr=uint32
  max_n_D : Product  Inputs=*/
  max_n_D1 : Product  Inputs=*/
  max_n_F : Constant  OutDataTypeStr=single
  max_n_L : simulink/Logic and Bit Operations/Bitwise Operator  logicop=AND  UseBitMask=on  BitMask=65535  BitMaskRealWorld=Stored Integer
  max_n_O : Constant  Value=0  OutDataTypeStr=single
  max_n_S : ArithShift
  max_n_sat : Saturate  UpperLimit=32767  LowerLimit=-32768
  max_n_st : Sum  Inputs=+-
  max_noutput4_C : Constant  Value=256
  max_nsubcon : Sum  Inputs=+-
  output1 : Outport
  output2 : Outport  Port=2
  output3 : Outport  Port=3
  output4 : Outport  Port=4
  output5 : Outport  Port=5
  output6 : Outport  Port=6
  output7 : Outport  Port=7
  output8 : Outport  Port=8
  wires:
  Constant8/1 -> output8/1
  Constant7/1 -> output7/1
  Constant6/1 -> output6/1
  Constant5/1 -> output5/1
  Constant2/1 -> output2/1
  Constant1/1 -> output1/1
  BitCov/1 -> output3/1
  max_n_And/1 -> BitCov/1
  max_n_And_C/1 -> max_n_And/2
  max_nCOV/1 -> output4/1
  max_n_D1/1 -> max_nCOV/1
  max_noutput4_C/1 -> max_n_D1/2
  max_n_L/1 -> max_n_And/1, max_n_D1/1
  max_n_Convert/1 -> max_n_L/1
  max_n_1sat/1 -> max_n_Convert/1
  max_n_S/1 -> max_n_1sat/1
  max_nSW/1 -> max_n_S/1
  max_nROP/1 -> max_nSW/2
  max_nsubcon/1 -> max_nSW/1
  max_nABS/1 -> max_nsubcon/2
  max_nCS/1 -> max_nsubcon/1
  max_nConS/1 -> max_nCS/1
  max_nCosR/1 -> max_nROP/2
  max_nRon/1 -> max_nSW/3, max_nABS/1, max_nROP/1
  max_n_D/1 -> max_nRon/1
  max_n_F/1 -> max_n_D/2
  max_n_st/1 -> max_n_D/1
  max_n_O/1 -> max_n_st/2
  max_n_sat/1 -> max_n_st/1
  max_n/1 -> max_n_sat/1

== system 21-E/run/ctrl/Subsystem/Subsystem ==
  In1 : Inport
  Saturation : Saturate  UpperLimit=2300  LowerLimit=0
  Switch : Switch
  Unit Delay : UnitDelay  SampleTime=-1
  Out1 : Outport
  wires:
  In1/1 -> Switch/1, Switch/2, Unit Delay/1
  Unit Delay/1 -> Switch/3
  Switch/1 -> Saturation/1
  Saturation/1 -> Out1/1

== system 21-E/run/ctrl/Subsystem1/Subsystem ==
  T1d : Inport
  T2d : Inport  Port=2
  Constant : Constant  Value=0.5
  Constant1 : Constant  Value=0.5
  Data Store Read1 : DataStoreRead  DataStoreName=Vture
  Data Store Read2 : DataStoreRead  DataStoreName=acc_signal
  Data Store Read3 : DataStoreRead  DataStoreName=Vture
  Data Type Conversion2 : DataTypeConversion  OutDataTypeStr=double
  Data Type Conversion3 : DataTypeConversion  OutDataTypeStr=double
  Gain : Gain  Gain=0.5
  Gain1 : Gain  Gain=1/0.0098
  Gain2 : Gain  Gain=1/0.0098
  Gain3 : Gain  Gain=1/12.5
  Gain4 : Gain  Gain=1/12.5
  Logical Operator : Logic  AllPortsSameDT=off  OutDataTypeStr=boolean
  MATLAB Function : MATLAB Function  TreatAsAtomicUnit=on
  Mux : Mux  Inputs=2
  Relational Operator : RelationalOperator  Operator=>  OutDataTypeStr=boolean
  Relational Operator1 : RelationalOperator  Operator=<=  OutDataTypeStr=boolean
  Subsystem : Subsystem
  Subsystem1 : Subsystem
  Switch : Switch  Criteria=u2 > Threshold
  T : Outport
  wires:
  Gain3/1 -> Gain1/1
  T1d/1 -> Gain3/1
  Gain2/1 -> Data Type Conversion3/1
  Gain1/1 -> Data Type Conversion2/1
  T2d/1 -> Gain4/1
  Gain4/1 -> Gain2/1
  Data Type Conversion2/1 -> Subsystem/1(In1)
  Data Type Conversion3/1 -> Subsystem1/1(In1)
  Data Store Read1/1 -> MATLAB Function/1(v)
  Subsystem/1(Out1) -> MATLAB Function/2(T1d)
  Subsystem1/1(Out1) -> MATLAB Function/3(T2d)
  Data Store Read2/1 -> Relational Operator/1
  Constant/1 -> Relational Operator/2
  Relational Operator/1 -> Logical Operator/1
  Data Store Read3/1 -> Relational Operator1/1
  Constant1/1 -> Relational Operator1/2
  Relational Operator1/1 -> Logical Operator/2
  Logical Operator/1 -> Switch/2
  MATLAB Function/1(T1) -> Mux/1
  MATLAB Function/2(T2) -> Mux/2
  Mux/1 -> Switch/3, Gain/1
  Gain/1 -> Switch/1
  Switch/1 -> T/1

== system 21-E/run/ctrl/Subsystem1/control ==
  k1 : Inport
  k2 : Inport  Port=2
  Data Store Write : DataStoreWrite  DataStoreName=slip_qian
  Data Store Write1 : DataStoreWrite  DataStoreName=slip_hou
  Subsystem : Subsystem
  Subsystem1 : Subsystem
  Subsystem2 : Subsystem
  Subsystem3 : Subsystem
  Subsystem4 : Subsystem
  Subsystem5 : Subsystem
  Subsystem6 : Subsystem
  T1 : Outport
  T2 : Outport  Port=2
  wires:
  Subsystem6/2(alp2d) -> [alp2]
  Subsystem/2(x2) -> [x2], Subsystem1/2(x2)
  Subsystem/1(x1) -> [x1], Subsystem1/1(x1)
  Subsystem/3(x3) -> Subsystem1/3(v)
  [phy1] -> Subsystem4/1(phy1)
  [alp1] -> Subsystem4/2(alp1)
  Subsystem6/1(alp1d) -> [alp1]
  Subsystem4/1(T1) -> T1/1
  k1/1 -> Subsystem6/5(k1)
  Subsystem3/1(W1) -> [w1]
  [phy2] -> Subsystem5/1(phy2)
  Subsystem2/2(phy2) -> [phy2]
  [x2] -> Subsystem6/2(x2)
  Subsystem3/2(W2) -> [w2]
  Subsystem2/1(phy1) -> [phy1]
  [x1] -> Subsystem6/1(x1)
  Subsystem1/2(s2) -> Data Store Write1/1, Subsystem2/2(s2)
  k2/1 -> Subsystem6/6(k2)
  Subsystem1/4(x4) -> Subsystem6/4(x4)
  Subsystem1/1(s1) -> Data Store Write/1, Subsystem2/1(s1)
  Subsystem1/3(x3) -> Subsystem6/3(x3)
  [alp2] -> Subsystem5/2(alp2)
  Subsystem5/1(T2) -> T2/1
  [w2] -> Subsystem5/3(W2)
  [w1] -> Subsystem4/3(W1)
  [phy1] -> Subsystem3/1(phy1)
  [phy2] -> Subsystem3/2(phy2)

== system 21-E/run/ctrl/Subsystem2/Subsystem ==
  In1 : Inport
  Saturation : Saturate  UpperLimit=2300  LowerLimit=0
  Switch : Switch  Criteria=u2 > Threshold
  Unit Delay : UnitDelay  SampleTime=-1
  Out1 : Outport
  wires:
  In1/1 -> Switch/1, Switch/2, Unit Delay/1
  Unit Delay/1 -> Switch/3
  Switch/1 -> Saturation/1
  Saturation/1 -> Out1/1

== system 21-E/run/ctrl/Subsystem2/Subsystem1 ==
  In1 : Inport
  Saturation : Saturate  UpperLimit=2300  LowerLimit=0
  Switch : Switch  Criteria=u2 > Threshold
  Unit Delay : UnitDelay  SampleTime=-1
  Out1 : Outport
  wires:
  Saturation/1 -> Out1/1
  Switch/1 -> Saturation/1
  Unit Delay/1 -> Switch/3
  In1/1 -> Unit Delay/1, Switch/2, Switch/1

== system 21-E/run/ctrl/amk_tpostive1/工况判断 ==
  note: 改中值！！！
  In1 : Inport
  In2 : Inport  Port=2
  In3 : Inport  Port=3
  In4 : Inport  Port=4
  In5 : Inport  Port=5
  In6 : Inport  Port=6
  In7 : Inport  Port=7
  In8 : Inport  Port=8
  Constant1 : Constant  Value=150
  Constant2 : Constant  Value=2742
  Constant3 : Constant  Value=150
  Constant4 : Constant  Value=1000
  Constant5 : Constant  Value=4514
  Data Store Read : DataStoreRead  DataStoreName=ANGLE
  Data Store Read1 : DataStoreRead  DataStoreName=ConditionJudge
  Data Store Read2 : DataStoreRead  DataStoreName=ANGLE_middle
  Data Store Read3 : DataStoreRead  DataStoreName=ANGLE_middle
  Data Store Write : DataStoreWrite  DataStoreName=ConditionJudge
  Data Store Write1 : DataStoreWrite  DataStoreName=ANGLE_middle
  Data Store Write2 : DataStoreWrite  DialogController=Simulink.DDGSource  DataStoreName=ANGLE_left
  Data Store Write3 : DataStoreWrite  DataStoreName=ANGLE_right
  Logical Operator : Logic  AllPortsSameDT=off  OutDataTypeStr=boolean
  Relational Operator : RelationalOperator  Operator=<=  OutDataTypeStr=boolean
  Relational Operator1 : RelationalOperator  Operator=<=  OutDataTypeStr=boolean
  Sum : Sum  Inputs=|+-
  Sum1 : Sum  Inputs=|++
  Switch{,1..3} (4 alike) : Switch  Criteria=u2 > Threshold
  Out1 : Outport
  Out2 : Outport  Port=2
  Out3 : Outport  Port=3
  Out4 : Outport  Port=4
  wires:
  Switch/1 -> Out1/1
  Switch2/1 -> Out3/1
  Switch3/1 -> Out4/1
  Switch1/1 -> Out2/1
  In2/1 -> Switch1/1
  In3/1 -> Switch2/1
  Data Store Read1/1 -> Switch3/2, Switch2/2, Switch/2, Switch1/2
  In1/1 -> Switch/1
  In5/1 -> Switch/3
  In4/1 -> Switch3/1
  In7/1 -> Switch2/3
  In8/1 -> Switch3/3
  In6/1 -> Switch1/3
  Sum1/1 -> Relational Operator/2
  Data Store Read/1 -> Relational Operator/1, Relational Operator1/2
  Sum/1 -> Relational Operator1/1
  Relational Operator1/1 -> Logical Operator/1
  Relational Operator/1 -> Logical Operator/2
  Logical Operator/1 -> Data Store Write/1
  Data Store Read2/1 -> Sum/1
  Constant3/1 -> Sum/2
  Data Store Read3/1 -> Sum1/1
  Constant1/1 -> Sum1/2
  Constant2/1 -> Data Store Write1/1
  Constant4/1 -> Data Store Write2/1
  Constant5/1 -> Data Store Write3/1

== system 21-E/run/ctrl/amk_tpostive1/差速 ==
  Data Store Read : DataStoreRead  DataStoreName=ANGLE
  Data Store Read1 : DataStoreRead  DataStoreName=Vture
  Data Store Read4 : DataStoreRead  DataStoreName=V3
  Data Store Read5 : DataStoreRead  DataStoreName=V4
  Subsystem1 : Subsystem
  Subsystem2 : Subsystem
  Out1 : Outport
  Out2 : Outport  Port=2
  Out3 : Outport  Port=3
  Out4 : Outport  Port=4
  wires:
  Data Store Read1/1 -> Subsystem2/1(vx)
  Data Store Read/1 -> Subsystem2/2(an)
  Subsystem2/1(vy) -> Subsystem1/1(vy)
  Subsystem2/3(ax) -> Subsystem1/3(ax)
  Subsystem2/4(ay) -> Subsystem1/4(ay)
  Subsystem2/2(yaw) -> Subsystem1/2(yaw)

== system 21-E/run/ctrl/amk_tpostive1/限滑 ==
  TP : Inport
  Data Store Write : DataStoreWrite  DataStoreName=slip_qian
  Data Store Write1 : DataStoreWrite  DataStoreName=slip_hou
  V前 : Subsystem
  V后 : Subsystem
  扭矩*PI1 : Subsystem
  扭矩*PI2 : Subsystem
  滑移率计算 : Subsystem
  滑移率计算1 : Subsystem
  Out1 : Outport
  Out2 : Outport  Port=2
  Out3 : Outport  Port=3
  Out4 : Outport  Port=4
  wires:
  滑移率计算/1(Out) -> 扭矩*PI1/2(滑移率输入), Data Store Write1/1  "slip2"
  V后/1(Out1) -> 滑移率计算/1(V后)  "vhou"
  扭矩*PI1/1(Out1) -> Out3/1, Out4/1
  TP/1 -> 扭矩*PI1/1(扭矩), 扭矩*PI2/2(扭矩)
  滑移率计算1/1(Out) -> 扭矩*PI2/1(滑移率输入), Data Store Write/1  "slip1"
  V前/1(Out1) -> 滑移率计算1/1(V前)  "vqian"
  扭矩*PI2/1(Out1) -> Out2/1, Out1/1

== system 21-E/run/ctrl/control/Subsystem ==
  Add : Sum
  Add1 : Sum
  Data Store Read : DataStoreRead  DataStoreName=V1
  Data Store Read1 : DataStoreRead  DataStoreName=V2
  Data Store Read2 : DataStoreRead  DataStoreName=V3
  Data Store Read3 : DataStoreRead  DataStoreName=V4
  Data Store Read4 : DataStoreRead  DataStoreName=Vture
  Gain : Gain  Gain=0.5
  Gain1 : Gain  Gain=0.5
  x1 : Outport
  x2 : Outport  Port=2
  x3 : Outport  Port=3
  wires:
  Gain/1 -> x1/1  "x1"
  Data Store Read4/1 -> x3/1  "x3"
  Data Store Read3/1 -> Add1/2
  Add/1 -> Gain/1
  Add1/1 -> Gain1/1
  Data Store Read2/1 -> Add1/1
  Data Store Read/1 -> Add/1
  Data Store Read1/1 -> Add/2
  Gain1/1 -> x2/1  "x2"

== system 21-E/run/ctrl/control/Subsystem1 ==
  x1 : Inport
  x2 : Inport  Port=2
  v : Inport  Port=3
  Add : Sum  Inputs=+-
  Add1 : Sum  Inputs=+-
  Constant : Constant
  Constant1 : Constant
  MATLAB Function : MATLAB Function  TreatAsAtomicUnit=on
  MATLAB Function1 : MATLAB Function  TreatAsAtomicUnit=on
  s1 : Outport
  s2 : Outport  Port=2
  x3 : Outport  Port=3
  x4 : Outport  Port=4
  wires:
  x2/1 -> MATLAB Function1/1(x)
  v/1 -> MATLAB Function1/2(v), MATLAB Function/2(v)
  x1/1 -> MATLAB Function/1(x)
  MATLAB Function/1(s) -> Add/2, s1/1
  MATLAB Function1/1(s) -> Add1/2, s2/1
  Constant/1 -> Add/1
  Add/1 -> x3/1
  Constant1/1 -> Add1/1
  Add1/1 -> x4/1

== system 21-E/run/ctrl/control/Subsystem2 ==
  s1 : Inport
  s2 : Inport  Port=2
  Constant : Constant  Value=0.01
  Constant1 : Constant  Value=0.01
  MATLAB Function : MATLAB Function  TreatAsAtomicUnit=on
  MATLAB Function1 : MATLAB Function  TreatAsAtomicUnit=on
  Switch : Switch  Criteria=u2 > Threshold
  Switch1 : Switch  Criteria=u2 > Threshold
  phy1 : Outport
  phy2 : Outport  Port=2
  wires:
  MATLAB Function1/1(phy) -> phy2/1
  MATLAB Function/1(phy) -> phy1/1
  s1/1 -> Switch/1, Switch/2
  Switch/1 -> MATLAB Function/1(s)
  Constant/1 -> Switch/3
  Switch1/1 -> MATLAB Function1/1(s)
  s2/1 -> Switch1/1, Switch1/2
  Constant1/1 -> Switch1/3

== system 21-E/run/ctrl/control/Subsystem3 ==
  phy1 : Inport
  phy2 : Inport  Port=2
  Add : Sum
  Add1 : Sum
  Data Store Read : DataStoreRead  DataStoreName=a
  Gain : Gain  Gain=0.5*9.8
  Gain1 : Gain  Gain=0.5
  L1 : Constant  Value=0.759
  L2 : Constant  Value=0.771
  M : Constant  Value=297
  MATLAB Function : MATLAB Function  TreatAsAtomicUnit=on
  Product : Product
  hg : Constant  Value=0.269
  W1 : Outport
  W2 : Outport  Port=2
  wires:
  L1/1 -> MATLAB Function/1(L1)
  Product/1 -> MATLAB Function/4(ah)
  MATLAB Function/2(W2) -> W2/1
  MATLAB Function/1(W1) -> W1/1
  L2/1 -> MATLAB Function/2(L2)
  M/1 -> MATLAB Function/3(M)
  hg/1 -> Product/1
  phy1/1 -> Add/1
  phy2/1 -> Add/2
  Add/1 -> Gain/1
  Gain/1 -> Add1/2
  Data Store Read/1 -> Add1/1
  Add1/1 -> Gain1/1
  Gain1/1 -> Product/2

== system 21-E/run/ctrl/control/Subsystem4 ==
  phy1 : Inport
  alp1 : Inport  Port=2
  W1 : Inport  Port=3
  Add : Sum
  Add1 : Sum
  Gain : Gain  Gain=0.225
  Gain1 : Gain  Gain=0.215
  Product : Product
  f1 : Constant  Value=0.01
  T1 : Outport
  wires:
  Add1/1 -> T1/1
  Gain1/1 -> Add1/2
  alp1/1 -> Gain1/1
  Product/1 -> Add1/1
  Add/1 -> Product/1
  f1/1 -> Add/1
  phy1/1 -> Add/2
  W1/1 -> Gain/1
  Gain/1 -> Product/2

== system 21-E/run/ctrl/control/Subsystem5 ==
  phy2 : Inport
  alp2 : Inport  Port=2
  W2 : Inport  Port=3
  Add : Sum
  Add1 : Sum
  Gain : Gain  Gain=0.225
  Gain1 : Gain  Gain=0.215
  Product : Product
  f2 : Constant  Value=0.01
  T2 : Outport
  wires:
  Gain/1 -> Product/2
  W2/1 -> Gain/1
  phy2/1 -> Add/2
  f2/1 -> Add/1
  Add/1 -> Product/1
  Product/1 -> Add1/1
  alp2/1 -> Gain1/1
  Gain1/1 -> Add1/2
  Add1/1 -> T2/1

== system 21-E/run/ctrl/control/Subsystem6 ==
  x1 : Inport
  x2 : Inport  Port=2
  x3 : Inport  Port=3
  x4 : Inport  Port=4
  k1 : Inport  Port=5
  k2 : Inport  Port=6
  Subsystem4 : Subsystem
  Subsystem5 : Subsystem
  alp1d : Outport
  alp2d : Outport  Port=2
  wires:
  Subsystem5/1(alp2d) -> alp2d/1
  x4/1 -> Subsystem5/2(x4)
  x2/1 -> Subsystem5/1(x2)
  k2/1 -> Subsystem5/3(k2)
  x3/1 -> Subsystem4/2(x3)
  k1/1 -> Subsystem4/3(k1)
  x1/1 -> Subsystem4/1(x1)
  Subsystem4/1(alp1d) -> alp1d/1

== system 21-E/run/ctrl/Subsystem1/Subsystem/Subsystem ==
  In1 : Inport
  Saturation : Saturate  UpperLimit=2300  LowerLimit=0
  Switch : Switch  Criteria=u2 > Threshold
  Unit Delay : UnitDelay  SampleTime=-1
  Out1 : Outport
  wires:
  In1/1 -> Switch/1, Switch/2, Unit Delay/1
  Unit Delay/1 -> Switch/3
  Switch/1 -> Saturation/1
  Saturation/1 -> Out1/1

== system 21-E/run/ctrl/Subsystem1/Subsystem/Subsystem1 ==
  In1 : Inport
  Saturation : Saturate  UpperLimit=2300  LowerLimit=0
  Switch : Switch  Criteria=u2 > Threshold
  Unit Delay : UnitDelay  SampleTime=-1
  Out1 : Outport
  wires:
  Saturation/1 -> Out1/1
  Switch/1 -> Saturation/1
  Unit Delay/1 -> Switch/3
  In1/1 -> Unit Delay/1, Switch/2, Switch/1

== system 21-E/run/ctrl/Subsystem1/control/Subsystem ==
  Add : Sum
  Add1 : Sum
  Data Store Read : DataStoreRead  DataStoreName=V1
  Data Store Read1 : DataStoreRead  DataStoreName=V2
  Data Store Read2 : DataStoreRead  DataStoreName=V3
  Data Store Read3 : DataStoreRead  DataStoreName=V4
  Data Store Read4 : DataStoreRead  DataStoreName=Vture
  Gain : Gain  Gain=0.5
  Gain1 : Gain  Gain=0.5
  x1 : Outport
  x2 : Outport  Port=2
  x3 : Outport  Port=3
  wires:
  Gain/1 -> x1/1  "x1"
  Data Store Read4/1 -> x3/1  "x3"
  Data Store Read3/1 -> Add1/2
  Add/1 -> Gain/1
  Add1/1 -> Gain1/1
  Data Store Read2/1 -> Add1/1
  Data Store Read/1 -> Add/1
  Data Store Read1/1 -> Add/2
  Gain1/1 -> x2/1  "x2"

== system 21-E/run/ctrl/Subsystem1/control/Subsystem1 ==
  x1 : Inport
  x2 : Inport  Port=2
  v : Inport  Port=3
  Add : Sum  Inputs=+-
  Add1 : Sum  Inputs=+-
  Constant : Constant
  Constant1 : Constant
  MATLAB Function : MATLAB Function  TreatAsAtomicUnit=on
  MATLAB Function1 : MATLAB Function  TreatAsAtomicUnit=on
  s1 : Outport
  s2 : Outport  Port=2
  x3 : Outport  Port=3
  x4 : Outport  Port=4
  wires:
  x2/1 -> MATLAB Function1/1(x)
  v/1 -> MATLAB Function1/2(v), MATLAB Function/2(v)
  x1/1 -> MATLAB Function/1(x)
  MATLAB Function/1(s) -> Add/2, s1/1
  MATLAB Function1/1(s) -> Add1/2, s2/1
  Constant/1 -> Add/1
  Add/1 -> x3/1
  Constant1/1 -> Add1/1
  Add1/1 -> x4/1

== system 21-E/run/ctrl/Subsystem1/control/Subsystem2 ==
  s1 : Inport
  s2 : Inport  Port=2
  Constant : Constant  Value=0.01
  Constant1 : Constant  Value=0.01
  MATLAB Function : MATLAB Function  TreatAsAtomicUnit=on
  MATLAB Function1 : MATLAB Function  TreatAsAtomicUnit=on
  Switch : Switch  Criteria=u2 > Threshold
  Switch1 : Switch  Criteria=u2 > Threshold
  phy1 : Outport
  phy2 : Outport  Port=2
  wires:
  MATLAB Function1/1(phy) -> phy2/1
  MATLAB Function/1(phy) -> phy1/1
  s1/1 -> Switch/1, Switch/2
  Switch/1 -> MATLAB Function/1(s)
  Constant/1 -> Switch/3
  Switch1/1 -> MATLAB Function1/1(s)
  s2/1 -> Switch1/1, Switch1/2
  Constant1/1 -> Switch1/3

== system 21-E/run/ctrl/Subsystem1/control/Subsystem3 ==
  phy1 : Inport
  phy2 : Inport  Port=2
  Add : Sum
  Add1 : Sum
  Data Store Read : DataStoreRead  DataStoreName=a
  Gain : Gain  Gain=0.5*9.8
  Gain1 : Gain  Gain=0.5
  L1 : Constant  Value=0.759
  L2 : Constant  Value=0.771
  M : Constant  Value=297
  MATLAB Function : MATLAB Function  TreatAsAtomicUnit=on
  Product : Product
  hg : Constant  Value=0.269
  W1 : Outport
  W2 : Outport  Port=2
  wires:
  L1/1 -> MATLAB Function/1(L1)
  Product/1 -> MATLAB Function/4(ah)
  MATLAB Function/2(W2) -> W2/1
  MATLAB Function/1(W1) -> W1/1
  L2/1 -> MATLAB Function/2(L2)
  M/1 -> MATLAB Function/3(M)
  hg/1 -> Product/1
  phy1/1 -> Add/1
  phy2/1 -> Add/2
  Add/1 -> Gain/1
  Gain/1 -> Add1/2
  Data Store Read/1 -> Add1/1
  Add1/1 -> Gain1/1
  Gain1/1 -> Product/2

== system 21-E/run/ctrl/Subsystem1/control/Subsystem4 ==
  phy1 : Inport
  alp1 : Inport  Port=2
  W1 : Inport  Port=3
  Add : Sum
  Add1 : Sum
  Gain : Gain  Gain=0.225
  Gain1 : Gain  Gain=0.215
  Product : Product
  f1 : Constant  Value=0.01
  T1 : Outport
  wires:
  Add1/1 -> T1/1
  Gain1/1 -> Add1/2
  alp1/1 -> Gain1/1
  Product/1 -> Add1/1
  Add/1 -> Product/1
  f1/1 -> Add/1
  phy1/1 -> Add/2
  W1/1 -> Gain/1
  Gain/1 -> Product/2

== system 21-E/run/ctrl/Subsystem1/control/Subsystem5 ==
  phy2 : Inport
  alp2 : Inport  Port=2
  W2 : Inport  Port=3
  Add : Sum
  Add1 : Sum
  Gain : Gain  Gain=0.225
  Gain1 : Gain  Gain=0.215
  Product : Product
  f2 : Constant  Value=0.01
  T2 : Outport
  wires:
  Gain/1 -> Product/2
  W2/1 -> Gain/1
  phy2/1 -> Add/2
  f2/1 -> Add/1
  Add/1 -> Product/1
  Product/1 -> Add1/1
  alp2/1 -> Gain1/1
  Gain1/1 -> Add1/2
  Add1/1 -> T2/1
